simulink model "BlockDiagram"  (R2021a)
settings: Solver=VariableStepAuto  StartTime=0.0  StopTime=10.0  RelTol=1e-3
values from neighbouring files (symbols this model uses):
  a = 0    [gainMaxDef.m]    (also in plot2.m = 2; simulink_test.m = 5)
  alpha = 1.195    [gainMaxDef.m]    (also in plot2.m = 1.9; simulink_test.m = 1.192)
  betac = 2    [plot2.m]    (also in simulink_test.m = 10)
  delay = 0.5    [plot2.m]    (also in simulink_test.m = 0.015)
  delay_a = 0.150    (= 0.15)    [plot2.m]    (also in simulink_test.m = 0.01)
  gnet = 40    [plot2.m]    (also in simulink_test.m = gnetset(k))
  omega = omegalist(l)    [gainMaxDef.m]    (also in plot2.m = 300; simulink_test.m = 0.8)
  omegader = 80    [simulink_test.m]
libraries: cstblocks x12
settings Model: Creator=shiva  LastModifiedBy=shiva

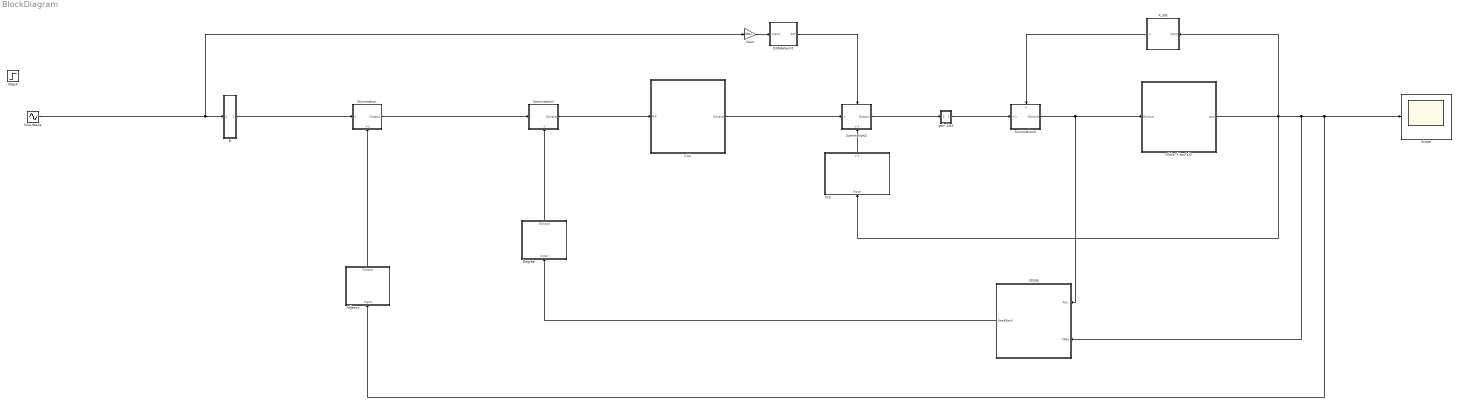
== system BlockDiagram ==
  Adjency : Subsystem
  B : Subsystem
  C(s) : Subsystem
  CDOB : Subsystem
  DSRdelayV2 : Subsystem
  Degree : Subsystem
  F(s) : Subsystem
  G(s)e^(-tau*s)2 : Subsystem
  Gain : Gain  Gain=betac
  Scope : Scope
  Sine Wave : Sin  SampleTime=0
  Step3 : Step  Time=0  SampleTime=0
  Summation : Subsystem
      settings: PortSchema="{\"entries\":[{\"content\":{\"sides\":[{\"content\":{\"connectorIds\":[\"In1\"]},\"type\":\"ConnectorPlacement.EquallySpacedRectSide\",\"uuid\":\"34a8278e-9c45-4ba9-8e7e-23ce47585cde\"},{\"content\":{\"connectorIds\":[\"Out1\"],\"side\":\"RIGHT\"},\"type\":\"ConnectorPlacement.EquallySpacedRectSide\",\"uuid\":\"649ea4d6-7388-43bb-a9cc-df912747b53e\"},{\"content\":{\"connectorIds\":[],\"side\":\"TOP\"},\"type\":\"ConnectorPlacement.EquallySpacedRectSide\",\"uuid\":\"5c1b8a35-4e2e-4e66-a4c8-170892603f16\"},{\"content\":{\"connectorIds\":[\"In2\"],\"side\":\"BOTTOM\"},\"type\":\"ConnectorPlacement.EquallySpacedRectSide\",\"uuid\":\"84c9cce4-2c6f-4c0c-8925-f02fa0e78f13\"}]},\"type\":\"ConnectorPlacement.EquallySpacedConnector\",\"uuid\":\"f49b62c2-1801-4f66-a651-2f339c5f1b03\"}],\"packageUris\":[\"http://schema.mathworks.com/mf0/Connector/R2020b\"],\"version\":\"1.0\"}"
  Summation1 : Subsystem
      settings: PortSchema="{\"entries\":[{\"content\":{\"sides\":[{\"content\":{\"connectorIds\":[\"In1\"]},\"type\":\"ConnectorPlacement.EquallySpacedRectSide\",\"uuid\":\"34a8278e-9c45-4ba9-8e7e-23ce47585cde\"},{\"content\":{\"connectorIds\":[\"Out1\"],\"side\":\"RIGHT\"},\"type\":\"ConnectorPlacement.EquallySpacedRectSide\",\"uuid\":\"649ea4d6-7388-43bb-a9cc-df912747b53e\"},{\"content\":{\"connectorIds\":[],\"side\":\"TOP\"},\"type\":\"ConnectorPlacement.EquallySpacedRectSide\",\"uuid\":\"5c1b8a35-4e2e-4e66-a4c8-170892603f16\"},{\"content\":{\"connectorIds\":[\"In2\"],\"side\":\"BOTTOM\"},\"type\":\"ConnectorPlacement.EquallySpacedRectSide\",\"uuid\":\"84c9cce4-2c6f-4c0c-8925-f02fa0e78f13\"}]},\"type\":\"ConnectorPlacement.EquallySpacedConnector\",\"uuid\":\"f49b62c2-1801-4f66-a651-2f339c5f1b03\"}],\"packageUris\":[\"http://schema.mathworks.com/mf0/Connector/R2020b\"],\"version\":\"1.0\"}"
  Summation2 : Subsystem
      settings: PortSchema="{\"entries\":[{\"content\":{\"sides\":[{\"content\":{\"connectorIds\":[\"In1\"]},\"type\":\"ConnectorPlacement.EquallySpacedRectSide\",\"uuid\":\"34a8278e-9c45-4ba9-8e7e-23ce47585cde\"},{\"content\":{\"connectorIds\":[\"Out1\"],\"side\":\"RIGHT\"},\"type\":\"ConnectorPlacement.EquallySpacedRectSide\",\"uuid\":\"649ea4d6-7388-43bb-a9cc-df912747b53e\"},{\"content\":{\"connectorIds\":[\"In2\"],\"side\":\"TOP\"},\"type\":\"ConnectorPlacement.EquallySpacedRectSide\",\"uuid\":\"5c1b8a35-4e2e-4e66-a4c8-170892603f16\"},{\"content\":{\"connectorIds\":[\"In3\"],\"side\":\"BOTTOM\"},\"type\":\"ConnectorPlacement.EquallySpacedRectSide\",\"uuid\":\"84c9cce4-2c6f-4c0c-8925-f02fa0e78f13\"}]},\"type\":\"ConnectorPlacement.EquallySpacedConnector\",\"uuid\":\"f49b62c2-1801-4f66-a651-2f339c5f1b03\"}],\"packageUris\":[\"http://schema.mathworks.com/mf0/Connector/R2020b\"],\"version\":\"1.0\"}"
  Summation3 : Subsystem
      settings: PortSchema="{\"entries\":[{\"content\":{\"sides\":[{\"content\":{\"connectorIds\":[\"In1\"]},\"type\":\"ConnectorPlacement.EquallySpacedRectSide\",\"uuid\":\"34a8278e-9c45-4ba9-8e7e-23ce47585cde\"},{\"content\":{\"connectorIds\":[\"Out1\"],\"side\":\"RIGHT\"},\"type\":\"ConnectorPlacement.EquallySpacedRectSide\",\"uuid\":\"649ea4d6-7388-43bb-a9cc-df912747b53e\"},{\"content\":{\"connectorIds\":[\"In2\"],\"side\":\"TOP\"},\"type\":\"ConnectorPlacement.EquallySpacedRectSide\",\"uuid\":\"5c1b8a35-4e2e-4e66-a4c8-170892603f16\"},{\"content\":{\"connectorIds\":[],\"side\":\"BOTTOM\"},\"type\":\"ConnectorPlacement.EquallySpacedRectSide\",\"uuid\":\"84c9cce4-2c6f-4c0c-8925-f02fa0e78f13\"}]},\"type\":\"ConnectorPlacement.EquallySpacedConnector\",\"uuid\":\"f49b62c2-1801-4f66-a651-2f339c5f1b03\"}],\"packageUris\":[\"http://schema.mathworks.com/mf0/Connector/R2020b\"],\"version\":\"1.0\"}"
  X_dot : Subsystem
  gain 1/a2 : Subsystem
  wires:
  Gain/1 -> DSRdelayV2/1(Input)
  Sine Wave/1 -> Gain/1, B/1(Input)
  G(s)e^(-tau*s)2/1(pos) -> F(s)/1(Input), CDOB/2(XRes), Adjency/1(Input), Scope/1, X_dot/1(Input)
  B/1(Output) -> Summation/1(+)
  gain 1/a2/1(u/a) -> Summation3/1(+1)
  X_dot/1(+) -> Summation3/2(+)
  Summation3/1(Output) -> CDOB/1(Acc.), G(s)e^(-tau*s)2/1(Output)
  Summation2/1(Output) -> gain 1/a2/1(u)
  F(s)/1(+1) -> Summation2/3(+1)
  DSRdelayV2/1(est) -> Summation2/2(-)
  C(s)/1(Output) -> Summation2/1(+)
  Summation1/1(Output) -> C(s)/1(R-F)
  Degree/1(Output) -> Summation1/2(+)
  Adjency/1(Output) -> Summation/2(+1)
  Summation/1(Output) -> Summation1/1(-)
  CDOB/1(FeedBack) -> Degree/1(Input)

== system BlockDiagram/Adjency ==
  Input : Inport
  Demux : Demux  Outputs=6
  Mux : Mux  Inputs=6
  Sum : Sum  Inputs=|++
  Sum1 : Sum  Inputs=|++
  Sum2 : Sum  Inputs=++++
  Terminator : Terminator
  Zero : Constant  Value=0  OutDataTypeStr=Inherit: Inherit via back propagation
  Output : Outport
  wires:
  Demux/2 -> Sum2/1, Mux/4, Sum1/2
  Demux/4 -> Sum2/3
  Demux/1 -> Sum1/1, Sum/1
  Sum1/1 -> Mux/3
  Zero/1 -> Mux/1
  Demux/6 -> Terminator/1
  Sum2/1 -> Mux/6
  Sum/1 -> Mux/2
  Demux/5 -> Sum2/4
  Demux/3 -> Sum/2, Mux/5, Sum2/2
  Input/1 -> Demux/1
  Mux/1 -> Output/1

== system BlockDiagram/B ==
  Input : Inport
  Mux : Mux  Inputs=6
  Zero : Constant  Value=0  OutDataTypeStr=Inherit: Inherit via back propagation
  Output : Outport
  wires:
  Input/1 -> Mux/1
  Zero/1 -> Mux/6, Mux/5, Mux/3, Mux/2, Mux/4
  Mux/1 -> Output/1

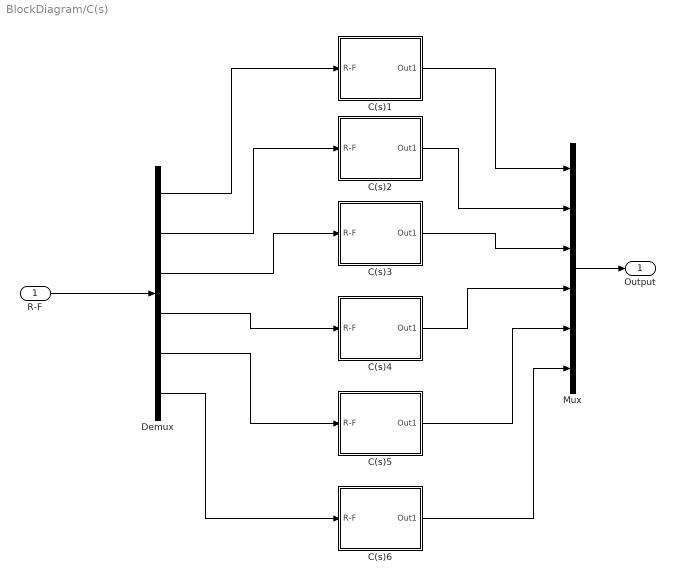
== system BlockDiagram/C(s) ==
  R-F : Inport
  C(s)1 : Subsystem
  C(s)2 : Subsystem
  C(s)3 : Subsystem
  C(s)4 : Subsystem
  C(s)5 : Subsystem
  C(s)6 : Subsystem
  Demux : Demux  Outputs=6
  Mux : Mux  Inputs=6
  Output : Outport
  wires:
  Demux/1 -> C(s)1/1(R-F)
  Demux/2 -> C(s)2/1(R-F)
  Demux/3 -> C(s)3/1(R-F)
  Demux/4 -> C(s)4/1(R-F)
  Demux/5 -> C(s)5/1(R-F)
  Demux/6 -> C(s)6/1(R-F)
  Mux/1 -> Output/1
  R-F/1 -> Demux/1
  C(s)1/1(Out1) -> Mux/1
  C(s)2/1(Out1) -> Mux/2
  C(s)3/1(Out1) -> Mux/3
  C(s)4/1(Out1) -> Mux/4
  C(s)5/1(Out1) -> Mux/5
  C(s)6/1(Out1) -> Mux/6

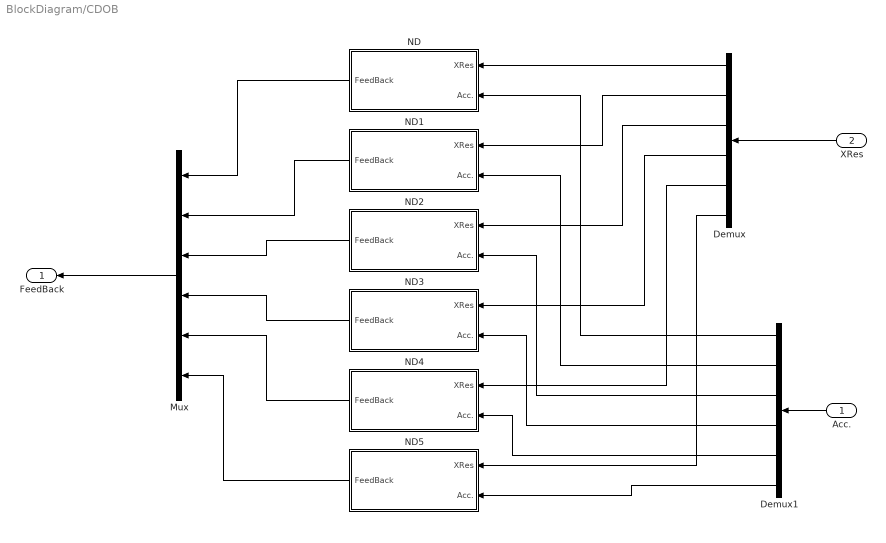
== system BlockDiagram/CDOB ==
  Acc. : Inport
  XRes : Inport  Port=2
  Demux : Demux  Outputs=6
  Demux1 : Demux  Outputs=6
  Mux : Mux  Inputs=6
  ND : Subsystem
  ND1 : Subsystem
  ND2 : Subsystem
  ND3 : Subsystem
  ND4 : Subsystem
  ND5 : Subsystem
  FeedBack : Outport
  wires:
  ND5/1(FeedBack) -> Mux/6
  ND1/1(FeedBack) -> Mux/2
  ND2/1(FeedBack) -> Mux/3
  ND4/1(FeedBack) -> Mux/5
  ND3/1(FeedBack) -> Mux/4
  ND/1(FeedBack) -> Mux/1
  Mux/1 -> FeedBack/1
  Demux/1 -> ND/1(XRes)
  Demux/2 -> ND1/1(XRes)
  Demux/3 -> ND2/1(XRes)
  Demux/4 -> ND3/1(XRes)
  Demux/5 -> ND4/1(XRes)
  Demux1/1 -> ND/2(Acc.)
  Demux1/2 -> ND1/2(Acc.)
  Demux1/3 -> ND2/2(Acc.)
  Demux1/4 -> ND3/2(Acc.)
  Demux1/5 -> ND4/2(Acc.)
  Acc./1 -> Demux1/1
  XRes/1 -> Demux/1
  Demux1/6 -> ND5/2(Acc.)
  Demux/6 -> ND5/1(XRes)

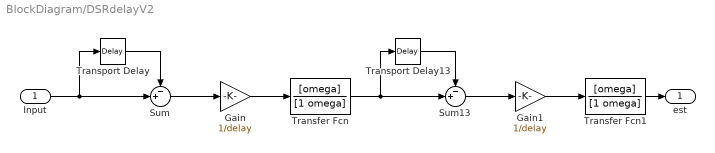
== system BlockDiagram/DSRdelayV2 ==
  Input : Inport
  Gain : Gain  Gain=1/delay
  Gain1 : Gain  Gain=1/delay
  Sum : Sum  Inputs=-+|
  Sum13 : Sum  Inputs=-+|
  Transfer Fcn : TransferFcn  Numerator=[omega]  Denominator=[1 omega]
  Transfer Fcn1 : TransferFcn  Numerator=[omega]  Denominator=[1 omega]
  Transport Delay : TransportDelay  DelayTime=delay
  Transport Delay13 : TransportDelay  DelayTime=delay
  est : Outport
  wires:
  Sum/1 -> Gain/1
  Gain/1 -> Transfer Fcn/1
  Transfer Fcn/1 -> Transport Delay13/1, Sum13/2
  Input/1 -> Transport Delay/1, Sum/2
  Transport Delay/1 -> Sum/1
  Transfer Fcn1/1 -> est/1
  Transport Delay13/1 -> Sum13/1
  Gain1/1 -> Transfer Fcn1/1
  Sum13/1 -> Gain1/1

== system BlockDiagram/Degree ==
  Input : Inport
  Demux : Demux  Outputs=6
  Gain : Gain  Gain=2
  Gain1 : Gain  Gain=2
  Gain4 : Gain  Gain=4
  Mux : Mux  Inputs=6
  Output : Outport
  wires:
  Gain1/1 -> Mux/3
  Demux/6 -> Gain4/1
  Gain4/1 -> Mux/6
  Gain/1 -> Mux/2
  Mux/1 -> Output/1
  Demux/1 -> Mux/1
  Demux/2 -> Gain/1
  Demux/3 -> Gain1/1
  Demux/4 -> Mux/4
  Demux/5 -> Mux/5
  Input/1 -> Demux/1

== system BlockDiagram/F(s) ==
  Input : Inport
  DSRdelayV1 : Subsystem
  DSRdelayV2 : Subsystem
  DSRdelayV3 : Subsystem
  DSRdelayV4 : Subsystem
  DSRdelayV5 : Subsystem
  DSRdelayV6 : Subsystem
  Demux : Demux  Outputs=6
  Mux : Mux  Inputs=6
  +1 : Outport
  wires:
  Input/1 -> Demux/1
  Mux/1 -> +1/1
  Demux/1 -> DSRdelayV2/1(Input)
  Demux/2 -> DSRdelayV1/1(Input)
  Demux/3 -> DSRdelayV3/1(Input)
  Demux/4 -> DSRdelayV4/1(Input)
  Demux/5 -> DSRdelayV5/1(Input)
  Demux/6 -> DSRdelayV6/1(Input)
  DSRdelayV2/1(est) -> Mux/1
  DSRdelayV1/1(est) -> Mux/2
  DSRdelayV3/1(est) -> Mux/3
  DSRdelayV4/1(est) -> Mux/4
  DSRdelayV5/1(est) -> Mux/5
  DSRdelayV6/1(est) -> Mux/6

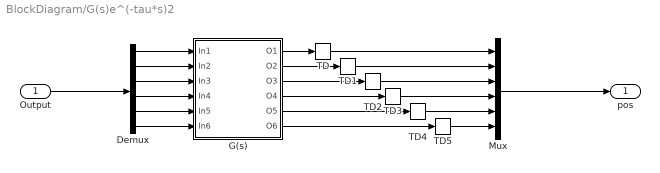
== system BlockDiagram/G(s)e^(-tau*s)2 ==
  Output : Inport
  Demux : Demux  Outputs=6
  G(s) : Subsystem
  Mux : Mux  Inputs=6
  TD{,1..5} (6 alike) : TransportDelay  DelayTime=delay_a
  pos : Outport
  wires:
  G(s)/3(O3) -> TD2/1
  G(s)/1(O1) -> TD/1
  G(s)/4(O4) -> TD3/1
  G(s)/5(O5) -> TD4/1
  G(s)/6(O6) -> TD5/1
  G(s)/2(O2) -> TD1/1
  Demux/1 -> G(s)/1(In1)
  Demux/2 -> G(s)/2(In2)
  Demux/3 -> G(s)/3(In3)
  Demux/4 -> G(s)/4(In4)
  Demux/5 -> G(s)/5(In5)
  Demux/6 -> G(s)/6(In6)
  Output/1 -> Demux/1
  TD/1 -> Mux/1
  Mux/1 -> pos/1
  TD1/1 -> Mux/2
  TD2/1 -> Mux/3
  TD3/1 -> Mux/4
  TD4/1 -> Mux/5
  TD5/1 -> Mux/6

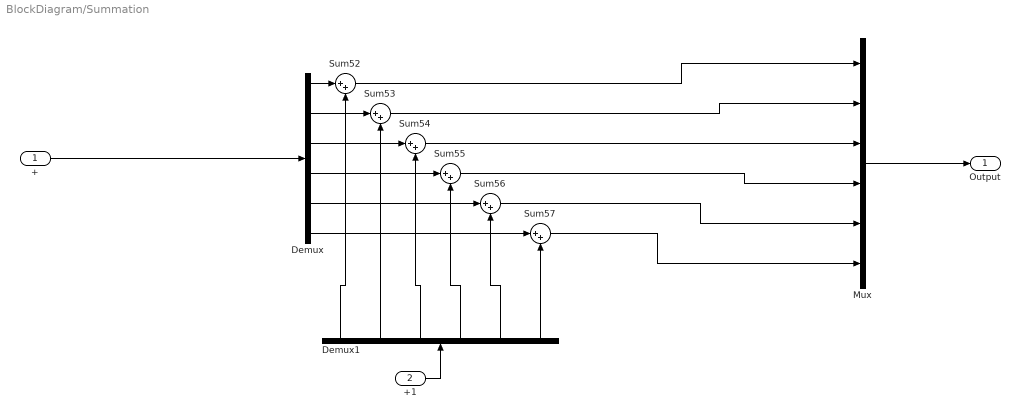
== system BlockDiagram/Summation ==
  + : Inport
  +1 : Inport  Port=2
  Demux : Demux  Outputs=6
  Demux1 : Demux  Outputs=6
  Mux : Mux  Inputs=6
  Sum{52..57} (6 alike) : Sum  Inputs=|++
  Output : Outport
  wires:
  Demux/3 -> Sum54/1
  Sum57/1 -> Mux/6
  Demux1/4 -> Sum55/2
  Demux/4 -> Sum55/1
  Sum56/1 -> Mux/5
  Demux/2 -> Sum53/1
  Demux1/1 -> Sum52/2
  Demux1/5 -> Sum56/2
  Demux1/6 -> Sum57/2
  Demux/6 -> Sum57/1
  Sum54/1 -> Mux/3
  Demux/5 -> Sum56/1
  Demux1/3 -> Sum54/2
  Demux/1 -> Sum52/1
  Demux1/2 -> Sum53/2
  +/1 -> Demux/1
  +1/1 -> Demux1/1
  Sum52/1 -> Mux/1
  Sum53/1 -> Mux/2
  Sum55/1 -> Mux/4
  Mux/1 -> Output/1

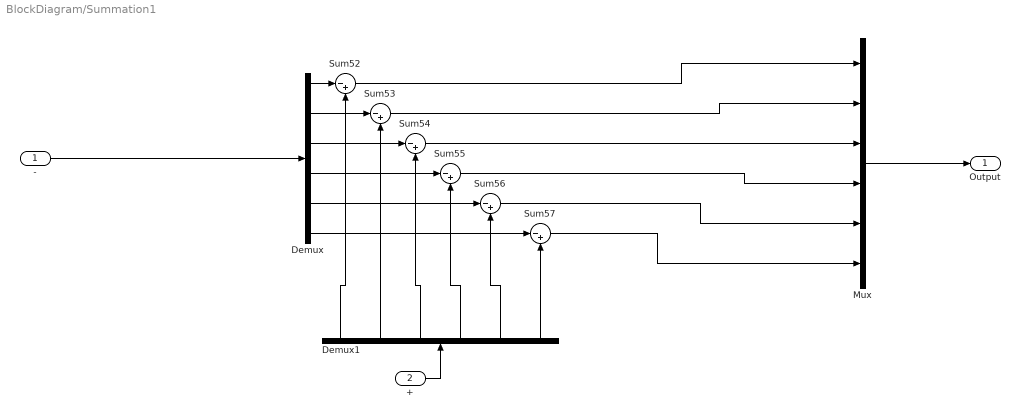
== system BlockDiagram/Summation1 ==
  - : Inport
  + : Inport  Port=2
  Demux : Demux  Outputs=6
  Demux1 : Demux  Outputs=6
  Mux : Mux  Inputs=6
  Sum{52..57} (6 alike) : Sum  Inputs=|-+
  Output : Outport
  wires:
  Demux/3 -> Sum54/1
  Sum57/1 -> Mux/6
  Demux1/4 -> Sum55/2
  Demux/4 -> Sum55/1
  Sum56/1 -> Mux/5
  Demux/2 -> Sum53/1
  Demux1/1 -> Sum52/2
  Demux1/5 -> Sum56/2
  Demux1/6 -> Sum57/2
  Demux/6 -> Sum57/1
  Sum54/1 -> Mux/3
  Demux/5 -> Sum56/1
  Demux1/3 -> Sum54/2
  Demux/1 -> Sum52/1
  Demux1/2 -> Sum53/2
  -/1 -> Demux/1
  +/1 -> Demux1/1
  Sum52/1 -> Mux/1
  Sum53/1 -> Mux/2
  Sum55/1 -> Mux/4
  Mux/1 -> Output/1

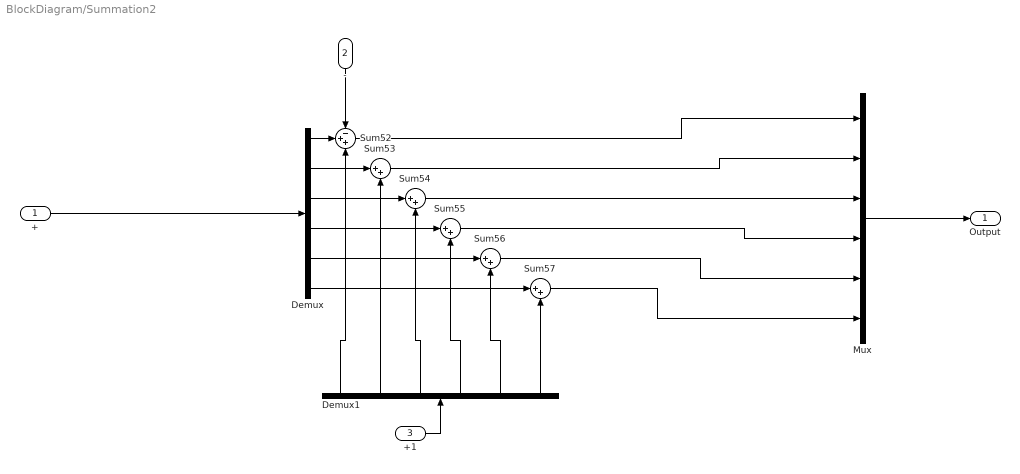
== system BlockDiagram/Summation2 ==
  + : Inport
  - : Inport  Port=2
  +1 : Inport  Port=3
  Demux : Demux  Outputs=6
  Demux1 : Demux  Outputs=6
  Mux : Mux  Inputs=6
  Sum52 : Sum  Inputs=-++
  Sum{53..57} (5 alike) : Sum  Inputs=|++
  Output : Outport
  wires:
  Demux/3 -> Sum54/1
  Sum57/1 -> Mux/6
  Demux1/4 -> Sum55/2
  Demux/4 -> Sum55/1
  Sum56/1 -> Mux/5
  Demux/2 -> Sum53/1
  Demux1/5 -> Sum56/2
  Demux1/6 -> Sum57/2
  Demux/6 -> Sum57/1
  Sum54/1 -> Mux/3
  Demux/5 -> Sum56/1
  Demux1/3 -> Sum54/2
  Demux1/2 -> Sum53/2
  +/1 -> Demux/1
  +1/1 -> Demux1/1
  Sum52/1 -> Mux/1
  Sum53/1 -> Mux/2
  Sum55/1 -> Mux/4
  Mux/1 -> Output/1
  Demux/1 -> Sum52/2
  -/1 -> Sum52/1
  Demux1/1 -> Sum52/3

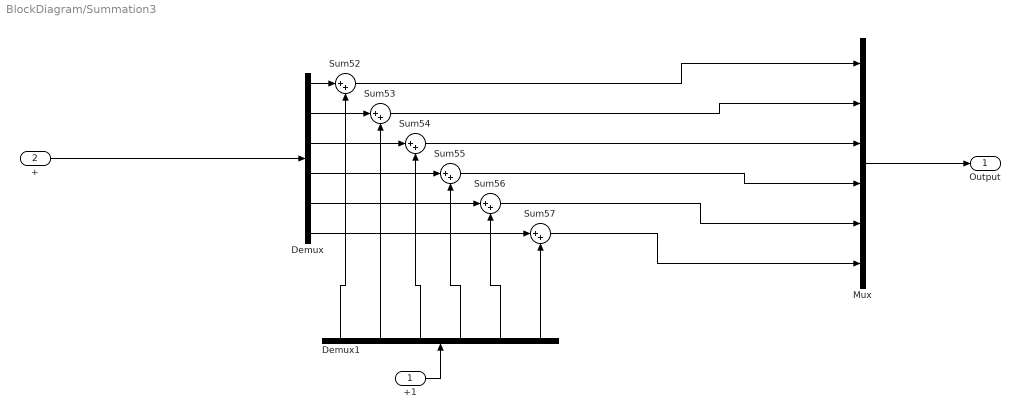
== system BlockDiagram/Summation3 ==
  +1 : Inport
  + : Inport  Port=2
  Demux : Demux  Outputs=6
  Demux1 : Demux  Outputs=6
  Mux : Mux  Inputs=6
  Sum{52..57} (6 alike) : Sum  Inputs=|++
  Output : Outport
  wires:
  Demux/3 -> Sum54/1
  Sum57/1 -> Mux/6
  Demux1/4 -> Sum55/2
  Demux/4 -> Sum55/1
  Sum56/1 -> Mux/5
  Demux/2 -> Sum53/1
  Demux1/1 -> Sum52/2
  Demux1/5 -> Sum56/2
  Demux1/6 -> Sum57/2
  Demux/6 -> Sum57/1
  Sum54/1 -> Mux/3
  Demux/5 -> Sum56/1
  Demux1/3 -> Sum54/2
  Demux/1 -> Sum52/1
  Demux1/2 -> Sum53/2
  +/1 -> Demux/1
  +1/1 -> Demux1/1
  Sum52/1 -> Mux/1
  Sum53/1 -> Mux/2
  Sum55/1 -> Mux/4
  Mux/1 -> Output/1

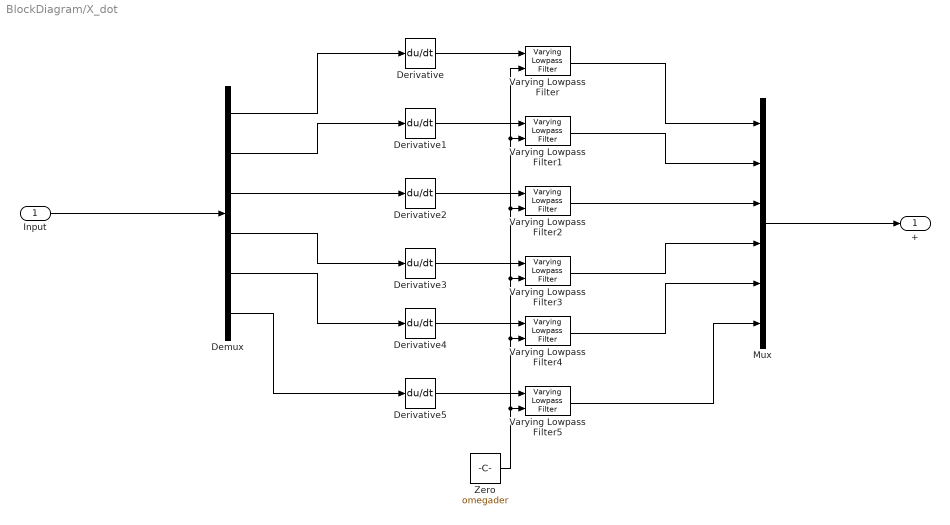
== system BlockDiagram/X_dot ==
  Input : Inport
  Demux : Demux  Outputs=6
  Derivative{,1..5} (6 alike) : Derivative
  Mux : Mux  Inputs=6
  Varying Lowpass Filter{,1..5} (6 alike) : cstblocks/Linear Parameter Varying/Varying Lowpass Filter  N=1
  Zero : Constant  Value=omegader  OutDataTypeStr=Inherit: Inherit via back propagation
  + : Outport
  wires:
  Derivative/1 -> Varying Lowpass Filter/1
  Derivative1/1 -> Varying Lowpass Filter1/1
  Derivative2/1 -> Varying Lowpass Filter2/1
  Derivative3/1 -> Varying Lowpass Filter3/1
  Derivative4/1 -> Varying Lowpass Filter4/1
  Derivative5/1 -> Varying Lowpass Filter5/1
  Zero/1 -> Varying Lowpass Filter3/2, Varying Lowpass Filter/2, Varying Lowpass Filter1/2, Varying Lowpass Filter2/2, Varying Lowpass Filter4/2, Varying Lowpass Filter5/2
  Input/1 -> Demux/1
  Demux/1 -> Derivative/1
  Demux/2 -> Derivative1/1
  Demux/3 -> Derivative2/1
  Demux/4 -> Derivative3/1
  Demux/5 -> Derivative4/1
  Demux/6 -> Derivative5/1
  Varying Lowpass Filter2/1 -> Mux/3
  Varying Lowpass Filter1/1 -> Mux/2
  Varying Lowpass Filter/1 -> Mux/1
  Varying Lowpass Filter3/1 -> Mux/4
  Varying Lowpass Filter4/1 -> Mux/5
  Varying Lowpass Filter5/1 -> Mux/6
  Mux/1 -> +/1

== system BlockDiagram/gain 1//a2 ==
  u : Inport
  1/a{,1..5} (6 alike) : Gain  Gain=1/a
  Demux : Demux  Outputs=6
  Mux : Mux  Inputs=6
  u/a : Outport
  wires:
  Mux/1 -> u/a/1
  u/1 -> Demux/1
  Demux/1 -> 1/a/1
  Demux/2 -> 1/a1/1
  Demux/3 -> 1/a2/1
  Demux/4 -> 1/a3/1
  Demux/5 -> 1/a4/1
  Demux/6 -> 1/a5/1
  1/a/1 -> Mux/1
  1/a1/1 -> Mux/2
  1/a2/1 -> Mux/3
  1/a3/1 -> Mux/4
  1/a4/1 -> Mux/5
  1/a5/1 -> Mux/6

== system BlockDiagram/C(s)/C(s)1 ==
  R-F : Inport
  DSRdelayV1 : Subsystem
  Derivative : Derivative
  Gain : Gain  Gain=betac
  Gain1 : Gain  Gain=betac*alpha^2
  Gain3 : Gain  Gain=2*alpha*betac
  Sum : Sum  Inputs=---
  Varying Lowpass Filter : cstblocks/Linear Parameter Varying/Varying Lowpass Filter  N=1
  Zero : Constant  Value=omegader  OutDataTypeStr=Inherit: Inherit via back propagation
  Out1 : Outport
  wires:
  Gain/1 -> DSRdelayV1/1(Input)
  Gain1/1 -> Sum/2
  Sum/1 -> Out1/1
  R-F/1 -> Gain3/1, Gain1/1, Gain/1
  DSRdelayV1/1(est) -> Sum/1
  Zero/1 -> Varying Lowpass Filter/2
  Varying Lowpass Filter/1 -> Sum/3
  Gain3/1 -> Derivative/1
  Derivative/1 -> Varying Lowpass Filter/1

== system BlockDiagram/C(s)/C(s)2 ==
  R-F : Inport
  DSRdelayV1 : Subsystem
  Derivative : Derivative
  Gain : Gain  Gain=betac
  Gain1 : Gain  Gain=betac*alpha^2
  Gain3 : Gain  Gain=2*alpha*betac
  Sum : Sum  Inputs=---
  Varying Lowpass Filter : cstblocks/Linear Parameter Varying/Varying Lowpass Filter  N=1
  Zero : Constant  Value=omegader  OutDataTypeStr=Inherit: Inherit via back propagation
  Out1 : Outport
  wires:
  Gain/1 -> DSRdelayV1/1(Input)
  Gain1/1 -> Sum/2
  Sum/1 -> Out1/1
  R-F/1 -> Gain3/1, Gain1/1, Gain/1
  DSRdelayV1/1(est) -> Sum/1
  Zero/1 -> Varying Lowpass Filter/2
  Varying Lowpass Filter/1 -> Sum/3
  Gain3/1 -> Derivative/1
  Derivative/1 -> Varying Lowpass Filter/1

== system BlockDiagram/C(s)/C(s)3 ==
  R-F : Inport
  DSRdelayV1 : Subsystem
  Derivative : Derivative
  Gain : Gain  Gain=betac
  Gain1 : Gain  Gain=betac*alpha^2
  Gain3 : Gain  Gain=2*alpha*betac
  Sum : Sum  Inputs=---
  Varying Lowpass Filter : cstblocks/Linear Parameter Varying/Varying Lowpass Filter  N=1
  Zero : Constant  Value=omegader  OutDataTypeStr=Inherit: Inherit via back propagation
  Out1 : Outport
  wires:
  Gain/1 -> DSRdelayV1/1(Input)
  Gain1/1 -> Sum/2
  Sum/1 -> Out1/1
  R-F/1 -> Gain3/1, Gain1/1, Gain/1
  DSRdelayV1/1(est) -> Sum/1
  Zero/1 -> Varying Lowpass Filter/2
  Varying Lowpass Filter/1 -> Sum/3
  Gain3/1 -> Derivative/1
  Derivative/1 -> Varying Lowpass Filter/1

== system BlockDiagram/C(s)/C(s)4 ==
  R-F : Inport
  DSRdelayV1 : Subsystem
  Derivative : Derivative
  Gain : Gain  Gain=betac
  Gain1 : Gain  Gain=betac*alpha^2
  Gain3 : Gain  Gain=2*alpha*betac
  Sum : Sum  Inputs=---
  Varying Lowpass Filter : cstblocks/Linear Parameter Varying/Varying Lowpass Filter  N=1
  Zero : Constant  Value=omegader  OutDataTypeStr=Inherit: Inherit via back propagation
  Out1 : Outport
  wires:
  Gain/1 -> DSRdelayV1/1(Input)
  Gain1/1 -> Sum/2
  Sum/1 -> Out1/1
  R-F/1 -> Gain3/1, Gain1/1, Gain/1
  DSRdelayV1/1(est) -> Sum/1
  Zero/1 -> Varying Lowpass Filter/2
  Varying Lowpass Filter/1 -> Sum/3
  Gain3/1 -> Derivative/1
  Derivative/1 -> Varying Lowpass Filter/1

== system BlockDiagram/C(s)/C(s)5 ==
  R-F : Inport
  DSRdelayV1 : Subsystem
  Derivative : Derivative
  Gain : Gain  Gain=betac
  Gain1 : Gain  Gain=betac*alpha^2
  Gain3 : Gain  Gain=2*alpha*betac
  Sum : Sum  Inputs=---
  Varying Lowpass Filter : cstblocks/Linear Parameter Varying/Varying Lowpass Filter  N=1
  Zero : Constant  Value=omegader  OutDataTypeStr=Inherit: Inherit via back propagation
  Out1 : Outport
  wires:
  Gain/1 -> DSRdelayV1/1(Input)
  Gain1/1 -> Sum/2
  Sum/1 -> Out1/1
  R-F/1 -> Gain3/1, Gain1/1, Gain/1
  DSRdelayV1/1(est) -> Sum/1
  Zero/1 -> Varying Lowpass Filter/2
  Varying Lowpass Filter/1 -> Sum/3
  Gain3/1 -> Derivative/1
  Derivative/1 -> Varying Lowpass Filter/1

== system BlockDiagram/C(s)/C(s)6 ==
  R-F : Inport
  DSRdelayV1 : Subsystem
  Derivative : Derivative
  Gain : Gain  Gain=betac
  Gain1 : Gain  Gain=betac*alpha^2
  Gain3 : Gain  Gain=2*alpha*betac
  Sum : Sum  Inputs=---
  Varying Lowpass Filter : cstblocks/Linear Parameter Varying/Varying Lowpass Filter  N=1
  Zero : Constant  Value=omegader  OutDataTypeStr=Inherit: Inherit via back propagation
  Out1 : Outport
  wires:
  Gain/1 -> DSRdelayV1/1(Input)
  Gain1/1 -> Sum/2
  Sum/1 -> Out1/1
  R-F/1 -> Gain3/1, Gain1/1, Gain/1
  DSRdelayV1/1(est) -> Sum/1
  Zero/1 -> Varying Lowpass Filter/2
  Varying Lowpass Filter/1 -> Sum/3
  Gain3/1 -> Derivative/1
  Derivative/1 -> Varying Lowpass Filter/1

== system BlockDiagram/CDOB/ND ==
  XRes : Inport
  Acc. : Inport  Port=2
  CDOB1 : Subsystem
  TimeDelayComp : Subsystem
  FeedBack : Outport
  wires:
  CDOB1/1(Dobsv) -> TimeDelayComp/2(Dobsv)
  Acc./1 -> CDOB1/2(Acc.)
  TimeDelayComp/1(FeedBack) -> FeedBack/1
  XRes/1 -> TimeDelayComp/1(SysOut), CDOB1/1(XRes)

== system BlockDiagram/CDOB/ND1 ==
  XRes : Inport
  Acc. : Inport  Port=2
  CDOB1 : Subsystem
  TimeDelayComp : Subsystem
  FeedBack : Outport
  wires:
  CDOB1/1(Dobsv) -> TimeDelayComp/2(Dobsv)
  Acc./1 -> CDOB1/2(Acc.)
  TimeDelayComp/1(FeedBack) -> FeedBack/1
  XRes/1 -> TimeDelayComp/1(SysOut), CDOB1/1(XRes)

== system BlockDiagram/CDOB/ND2 ==
  XRes : Inport
  Acc. : Inport  Port=2
  CDOB1 : Subsystem
  TimeDelayComp : Subsystem
  FeedBack : Outport
  wires:
  CDOB1/1(Dobsv) -> TimeDelayComp/2(Dobsv)
  Acc./1 -> CDOB1/2(Acc.)
  TimeDelayComp/1(FeedBack) -> FeedBack/1
  XRes/1 -> TimeDelayComp/1(SysOut), CDOB1/1(XRes)

== system BlockDiagram/CDOB/ND3 ==
  XRes : Inport
  Acc. : Inport  Port=2
  CDOB1 : Subsystem
  TimeDelayComp : Subsystem
  FeedBack : Outport
  wires:
  CDOB1/1(Dobsv) -> TimeDelayComp/2(Dobsv)
  Acc./1 -> CDOB1/2(Acc.)
  TimeDelayComp/1(FeedBack) -> FeedBack/1
  XRes/1 -> TimeDelayComp/1(SysOut), CDOB1/1(XRes)

== system BlockDiagram/CDOB/ND4 ==
  XRes : Inport
  Acc. : Inport  Port=2
  CDOB1 : Subsystem
  TimeDelayComp : Subsystem
  FeedBack : Outport
  wires:
  CDOB1/1(Dobsv) -> TimeDelayComp/2(Dobsv)
  Acc./1 -> CDOB1/2(Acc.)
  TimeDelayComp/1(FeedBack) -> FeedBack/1
  XRes/1 -> TimeDelayComp/1(SysOut), CDOB1/1(XRes)

== system BlockDiagram/CDOB/ND5 ==
  XRes : Inport
  Acc. : Inport  Port=2
  CDOB1 : Subsystem
  TimeDelayComp : Subsystem
  FeedBack : Outport
  wires:
  CDOB1/1(Dobsv) -> TimeDelayComp/2(Dobsv)
  Acc./1 -> CDOB1/2(Acc.)
  TimeDelayComp/1(FeedBack) -> FeedBack/1
  XRes/1 -> TimeDelayComp/1(SysOut), CDOB1/1(XRes)

== system BlockDiagram/F(s)/DSRdelayV1 ==
  Input : Inport
  Gain : Gain  Gain=1/delay
  Gain1 : Gain  Gain=1/delay
  Sum : Sum  Inputs=-+|
  Sum13 : Sum  Inputs=-+|
  Transfer Fcn : TransferFcn  Numerator=[omega]  Denominator=[1 omega]
  Transfer Fcn1 : TransferFcn  Numerator=[omega]  Denominator=[1 omega]
  Transport Delay : TransportDelay  DelayTime=delay
  Transport Delay13 : TransportDelay  DelayTime=delay
  est : Outport
  wires:
  Sum/1 -> Gain/1
  Gain/1 -> Transfer Fcn/1
  Transfer Fcn/1 -> Transport Delay13/1, Sum13/2
  Input/1 -> Transport Delay/1, Sum/2
  Transport Delay/1 -> Sum/1
  Transfer Fcn1/1 -> est/1
  Transport Delay13/1 -> Sum13/1
  Gain1/1 -> Transfer Fcn1/1
  Sum13/1 -> Gain1/1

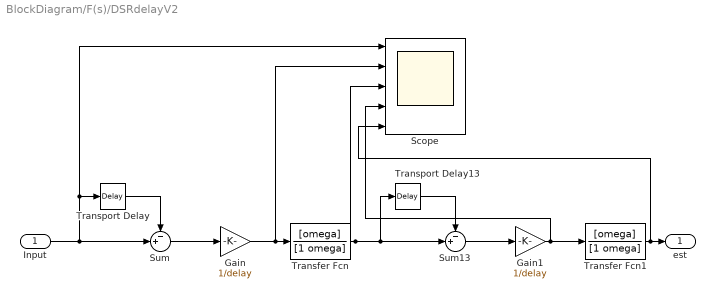
== system BlockDiagram/F(s)/DSRdelayV2 ==
  Input : Inport
  Gain : Gain  Gain=1/delay
  Gain1 : Gain  Gain=1/delay
  Scope : Scope  NumInputPorts=5
  Sum : Sum  Inputs=-+|
  Sum13 : Sum  Inputs=-+|
  Transfer Fcn : TransferFcn  Numerator=[omega]  Denominator=[1 omega]
  Transfer Fcn1 : TransferFcn  Numerator=[omega]  Denominator=[1 omega]
  Transport Delay : TransportDelay  DelayTime=delay
  Transport Delay13 : TransportDelay  DelayTime=delay
  est : Outport
  wires:
  Sum/1 -> Gain/1
  Gain/1 -> Scope/2, Transfer Fcn/1
  Transfer Fcn/1 -> Transport Delay13/1, Sum13/2, Scope/3
  Input/1 -> Transport Delay/1, Scope/1, Sum/2
  Transport Delay/1 -> Sum/1
  Transfer Fcn1/1 -> Scope/5, est/1
  Transport Delay13/1 -> Sum13/1
  Gain1/1 -> Scope/4, Transfer Fcn1/1
  Sum13/1 -> Gain1/1

== system BlockDiagram/F(s)/DSRdelayV3 ==
  Input : Inport
  Gain : Gain  Gain=1/delay
  Gain1 : Gain  Gain=1/delay
  Sum : Sum  Inputs=-+|
  Sum13 : Sum  Inputs=-+|
  Transfer Fcn : TransferFcn  Numerator=[omega]  Denominator=[1 omega]
  Transfer Fcn1 : TransferFcn  Numerator=[omega]  Denominator=[1 omega]
  Transport Delay : TransportDelay  DelayTime=delay
  Transport Delay13 : TransportDelay  DelayTime=delay
  est : Outport
  wires:
  Sum/1 -> Gain/1
  Gain/1 -> Transfer Fcn/1
  Transfer Fcn/1 -> Transport Delay13/1, Sum13/2
  Input/1 -> Transport Delay/1, Sum/2
  Transport Delay/1 -> Sum/1
  Transfer Fcn1/1 -> est/1
  Transport Delay13/1 -> Sum13/1
  Gain1/1 -> Transfer Fcn1/1
  Sum13/1 -> Gain1/1

== system BlockDiagram/F(s)/DSRdelayV4 ==
  Input : Inport
  Gain : Gain  Gain=1/delay
  Gain1 : Gain  Gain=1/delay
  Sum : Sum  Inputs=-+|
  Sum13 : Sum  Inputs=-+|
  Transfer Fcn : TransferFcn  Numerator=[omega]  Denominator=[1 omega]
  Transfer Fcn1 : TransferFcn  Numerator=[omega]  Denominator=[1 omega]
  Transport Delay : TransportDelay  DelayTime=delay
  Transport Delay13 : TransportDelay  DelayTime=delay
  est : Outport
  wires:
  Sum/1 -> Gain/1
  Gain/1 -> Transfer Fcn/1
  Transfer Fcn/1 -> Transport Delay13/1, Sum13/2
  Input/1 -> Transport Delay/1, Sum/2
  Transport Delay/1 -> Sum/1
  Transfer Fcn1/1 -> est/1
  Transport Delay13/1 -> Sum13/1
  Gain1/1 -> Transfer Fcn1/1
  Sum13/1 -> Gain1/1

== system BlockDiagram/F(s)/DSRdelayV5 ==
  Input : Inport
  Gain : Gain  Gain=1/delay
  Gain1 : Gain  Gain=1/delay
  Sum : Sum  Inputs=-+|
  Sum13 : Sum  Inputs=-+|
  Transfer Fcn : TransferFcn  Numerator=[omega]  Denominator=[1 omega]
  Transfer Fcn1 : TransferFcn  Numerator=[omega]  Denominator=[1 omega]
  Transport Delay : TransportDelay  DelayTime=delay
  Transport Delay13 : TransportDelay  DelayTime=delay
  est : Outport
  wires:
  Sum/1 -> Gain/1
  Gain/1 -> Transfer Fcn/1
  Transfer Fcn/1 -> Transport Delay13/1, Sum13/2
  Input/1 -> Transport Delay/1, Sum/2
  Transport Delay/1 -> Sum/1
  Transfer Fcn1/1 -> est/1
  Transport Delay13/1 -> Sum13/1
  Gain1/1 -> Transfer Fcn1/1
  Sum13/1 -> Gain1/1

== system BlockDiagram/F(s)/DSRdelayV6 ==
  Input : Inport
  Gain : Gain  Gain=1/delay
  Gain1 : Gain  Gain=1/delay
  Sum : Sum  Inputs=-+|
  Sum13 : Sum  Inputs=-+|
  Transfer Fcn : TransferFcn  Numerator=[omega]  Denominator=[1 omega]
  Transfer Fcn1 : TransferFcn  Numerator=[omega]  Denominator=[1 omega]
  Transport Delay : TransportDelay  DelayTime=delay
  Transport Delay13 : TransportDelay  DelayTime=delay
  est : Outport
  wires:
  Sum/1 -> Gain/1
  Gain/1 -> Transfer Fcn/1
  Transfer Fcn/1 -> Transport Delay13/1, Sum13/2
  Input/1 -> Transport Delay/1, Sum/2
  Transport Delay/1 -> Sum/1
  Transfer Fcn1/1 -> est/1
  Transport Delay13/1 -> Sum13/1
  Gain1/1 -> Transfer Fcn1/1
  Sum13/1 -> Gain1/1

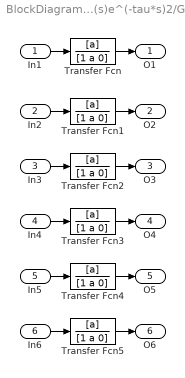
== system BlockDiagram/G(s)e^(-tau*s)2/G(s) ==
  In1 : Inport
  In2 : Inport  Port=2
  In3 : Inport  Port=3
  In4 : Inport  Port=4
  In5 : Inport  Port=5
  In6 : Inport  Port=6
  Transfer Fcn{,1..5} (6 alike) : TransferFcn  Numerator=[a]  Denominator=[1 a 0]
  O1 : Outport
  O2 : Outport  Port=2
  O3 : Outport  Port=3
  O4 : Outport  Port=4
  O5 : Outport  Port=5
  O6 : Outport  Port=6
  wires:
  Transfer Fcn1/1 -> O2/1
  In1/1 -> Transfer Fcn/1
  Transfer Fcn/1 -> O1/1
  In4/1 -> Transfer Fcn3/1
  Transfer Fcn3/1 -> O4/1
  In3/1 -> Transfer Fcn2/1
  In2/1 -> Transfer Fcn1/1
  Transfer Fcn2/1 -> O3/1
  Transfer Fcn5/1 -> O6/1
  In6/1 -> Transfer Fcn5/1
  In5/1 -> Transfer Fcn4/1
  Transfer Fcn4/1 -> O5/1

== system BlockDiagram/C(s)/C(s)1/DSRdelayV1 ==
  Input : Inport
  Gain : Gain  Gain=1/delay
  Gain1 : Gain  Gain=1/delay
  Sum : Sum  Inputs=-+|
  Sum13 : Sum  Inputs=-+|
  Transfer Fcn : TransferFcn  Numerator=[omega]  Denominator=[1 omega]
  Transfer Fcn1 : TransferFcn  Numerator=[omega]  Denominator=[1 omega]
  Transport Delay : TransportDelay  DelayTime=delay
  Transport Delay13 : TransportDelay  DelayTime=delay
  est : Outport
  wires:
  Sum/1 -> Gain/1
  Gain/1 -> Transfer Fcn/1
  Transfer Fcn/1 -> Transport Delay13/1, Sum13/2
  Input/1 -> Transport Delay/1, Sum/2
  Transport Delay/1 -> Sum/1
  Transfer Fcn1/1 -> est/1
  Transport Delay13/1 -> Sum13/1
  Gain1/1 -> Transfer Fcn1/1
  Sum13/1 -> Gain1/1

== system BlockDiagram/C(s)/C(s)2/DSRdelayV1 ==
  Input : Inport
  Gain : Gain  Gain=1/delay
  Gain1 : Gain  Gain=1/delay
  Sum : Sum  Inputs=-+|
  Sum13 : Sum  Inputs=-+|
  Transfer Fcn : TransferFcn  Numerator=[omega]  Denominator=[1 omega]
  Transfer Fcn1 : TransferFcn  Numerator=[omega]  Denominator=[1 omega]
  Transport Delay : TransportDelay  DelayTime=delay
  Transport Delay13 : TransportDelay  DelayTime=delay
  est : Outport
  wires:
  Sum/1 -> Gain/1
  Gain/1 -> Transfer Fcn/1
  Transfer Fcn/1 -> Transport Delay13/1, Sum13/2
  Input/1 -> Transport Delay/1, Sum/2
  Transport Delay/1 -> Sum/1
  Transfer Fcn1/1 -> est/1
  Transport Delay13/1 -> Sum13/1
  Gain1/1 -> Transfer Fcn1/1
  Sum13/1 -> Gain1/1

== system BlockDiagram/C(s)/C(s)3/DSRdelayV1 ==
  Input : Inport
  Gain : Gain  Gain=1/delay
  Gain1 : Gain  Gain=1/delay
  Sum : Sum  Inputs=-+|
  Sum13 : Sum  Inputs=-+|
  Transfer Fcn : TransferFcn  Numerator=[omega]  Denominator=[1 omega]
  Transfer Fcn1 : TransferFcn  Numerator=[omega]  Denominator=[1 omega]
  Transport Delay : TransportDelay  DelayTime=delay
  Transport Delay13 : TransportDelay  DelayTime=delay
  est : Outport
  wires:
  Sum/1 -> Gain/1
  Gain/1 -> Transfer Fcn/1
  Transfer Fcn/1 -> Transport Delay13/1, Sum13/2
  Input/1 -> Transport Delay/1, Sum/2
  Transport Delay/1 -> Sum/1
  Transfer Fcn1/1 -> est/1
  Transport Delay13/1 -> Sum13/1
  Gain1/1 -> Transfer Fcn1/1
  Sum13/1 -> Gain1/1

== system BlockDiagram/C(s)/C(s)4/DSRdelayV1 ==
  Input : Inport
  Gain : Gain  Gain=1/delay
  Gain1 : Gain  Gain=1/delay
  Sum : Sum  Inputs=-+|
  Sum13 : Sum  Inputs=-+|
  Transfer Fcn : TransferFcn  Numerator=[omega]  Denominator=[1 omega]
  Transfer Fcn1 : TransferFcn  Numerator=[omega]  Denominator=[1 omega]
  Transport Delay : TransportDelay  DelayTime=delay
  Transport Delay13 : TransportDelay  DelayTime=delay
  est : Outport
  wires:
  Sum/1 -> Gain/1
  Gain/1 -> Transfer Fcn/1
  Transfer Fcn/1 -> Transport Delay13/1, Sum13/2
  Input/1 -> Transport Delay/1, Sum/2
  Transport Delay/1 -> Sum/1
  Transfer Fcn1/1 -> est/1
  Transport Delay13/1 -> Sum13/1
  Gain1/1 -> Transfer Fcn1/1
  Sum13/1 -> Gain1/1

== system BlockDiagram/C(s)/C(s)5/DSRdelayV1 ==
  Input : Inport
  Gain : Gain  Gain=1/delay
  Gain1 : Gain  Gain=1/delay
  Sum : Sum  Inputs=-+|
  Sum13 : Sum  Inputs=-+|
  Transfer Fcn : TransferFcn  Numerator=[omega]  Denominator=[1 omega]
  Transfer Fcn1 : TransferFcn  Numerator=[omega]  Denominator=[1 omega]
  Transport Delay : TransportDelay  DelayTime=delay
  Transport Delay13 : TransportDelay  DelayTime=delay
  est : Outport
  wires:
  Sum/1 -> Gain/1
  Gain/1 -> Transfer Fcn/1
  Transfer Fcn/1 -> Transport Delay13/1, Sum13/2
  Input/1 -> Transport Delay/1, Sum/2
  Transport Delay/1 -> Sum/1
  Transfer Fcn1/1 -> est/1
  Transport Delay13/1 -> Sum13/1
  Gain1/1 -> Transfer Fcn1/1
  Sum13/1 -> Gain1/1

== system BlockDiagram/C(s)/C(s)6/DSRdelayV1 ==
  Input : Inport
  Gain : Gain  Gain=1/delay
  Gain1 : Gain  Gain=1/delay
  Sum : Sum  Inputs=-+|
  Sum13 : Sum  Inputs=-+|
  Transfer Fcn : TransferFcn  Numerator=[omega]  Denominator=[1 omega]
  Transfer Fcn1 : TransferFcn  Numerator=[omega]  Denominator=[1 omega]
  Transport Delay : TransportDelay  DelayTime=delay
  Transport Delay13 : TransportDelay  DelayTime=delay
  est : Outport
  wires:
  Sum/1 -> Gain/1
  Gain/1 -> Transfer Fcn/1
  Transfer Fcn/1 -> Transport Delay13/1, Sum13/2
  Input/1 -> Transport Delay/1, Sum/2
  Transport Delay/1 -> Sum/1
  Transfer Fcn1/1 -> est/1
  Transport Delay13/1 -> Sum13/1
  Gain1/1 -> Transfer Fcn1/1
  Sum13/1 -> Gain1/1

== system BlockDiagram/CDOB/ND/CDOB1 ==
  XRes : Inport
  Acc. : Inport  Port=2
  Derivative : Derivative  CoefficientInTFapproximation=0
  Gain : Gain  Gain=gnet/a
  Sum : Sum  Inputs=-+|
  Sum8 : Sum  Inputs=+-+
  Transfer Fcn2 : TransferFcn  Numerator=[gnet]  Denominator=[1 gnet]
  Dobsv : Outport
  wires:
  Transfer Fcn2/1 -> Sum/2
  Sum8/1 -> Transfer Fcn2/1
  Derivative/1 -> Sum8/2, Gain/1
  Gain/1 -> Sum8/1, Sum/1
  Sum/1 -> Dobsv/1
  XRes/1 -> Derivative/1
  Acc./1 -> Sum8/3

== system BlockDiagram/CDOB/ND/TimeDelayComp ==
  SysOut : Inport
  Dobsv : Inport  Port=2
  DelayCom : TransferFcn  Numerator=[a]  Denominator=[1 a 0]
  Sum8 : Sum  Inputs=|++
  FeedBack : Outport
  wires:
  DelayCom/1 -> Sum8/2
  SysOut/1 -> Sum8/1
  Sum8/1 -> FeedBack/1
  Dobsv/1 -> DelayCom/1

== system BlockDiagram/CDOB/ND1/CDOB1 ==
  XRes : Inport
  Acc. : Inport  Port=2
  Derivative : Derivative  CoefficientInTFapproximation=0
  Gain : Gain  Gain=gnet/a
  Sum : Sum  Inputs=-+|
  Sum8 : Sum  Inputs=+-+
  Transfer Fcn2 : TransferFcn  Numerator=[gnet]  Denominator=[1 gnet]
  Dobsv : Outport
  wires:
  Transfer Fcn2/1 -> Sum/2
  Sum8/1 -> Transfer Fcn2/1
  Derivative/1 -> Sum8/2, Gain/1
  Gain/1 -> Sum8/1, Sum/1
  Sum/1 -> Dobsv/1
  XRes/1 -> Derivative/1
  Acc./1 -> Sum8/3

== system BlockDiagram/CDOB/ND1/TimeDelayComp ==
  SysOut : Inport
  Dobsv : Inport  Port=2
  DelayCom : TransferFcn  Numerator=[a]  Denominator=[1 a 0]
  Sum8 : Sum  Inputs=|++
  FeedBack : Outport
  wires:
  DelayCom/1 -> Sum8/2
  SysOut/1 -> Sum8/1
  Sum8/1 -> FeedBack/1
  Dobsv/1 -> DelayCom/1

== system BlockDiagram/CDOB/ND2/CDOB1 ==
  XRes : Inport
  Acc. : Inport  Port=2
  Derivative : Derivative  CoefficientInTFapproximation=0
  Gain : Gain  Gain=gnet/a
  Sum : Sum  Inputs=-+|
  Sum8 : Sum  Inputs=+-+
  Transfer Fcn2 : TransferFcn  Numerator=[gnet]  Denominator=[1 gnet]
  Dobsv : Outport
  wires:
  Transfer Fcn2/1 -> Sum/2
  Sum8/1 -> Transfer Fcn2/1
  Derivative/1 -> Sum8/2, Gain/1
  Gain/1 -> Sum8/1, Sum/1
  Sum/1 -> Dobsv/1
  XRes/1 -> Derivative/1
  Acc./1 -> Sum8/3

== system BlockDiagram/CDOB/ND2/TimeDelayComp ==
  SysOut : Inport
  Dobsv : Inport  Port=2
  DelayCom : TransferFcn  Numerator=[a]  Denominator=[1 a 0]
  Sum8 : Sum  Inputs=|++
  FeedBack : Outport
  wires:
  DelayCom/1 -> Sum8/2
  SysOut/1 -> Sum8/1
  Sum8/1 -> FeedBack/1
  Dobsv/1 -> DelayCom/1

== system BlockDiagram/CDOB/ND3/CDOB1 ==
  XRes : Inport
  Acc. : Inport  Port=2
  Derivative : Derivative  CoefficientInTFapproximation=0
  Gain : Gain  Gain=gnet/a
  Sum : Sum  Inputs=-+|
  Sum8 : Sum  Inputs=+-+
  Transfer Fcn2 : TransferFcn  Numerator=[gnet]  Denominator=[1 gnet]
  Dobsv : Outport
  wires:
  Transfer Fcn2/1 -> Sum/2
  Sum8/1 -> Transfer Fcn2/1
  Derivative/1 -> Sum8/2, Gain/1
  Gain/1 -> Sum8/1, Sum/1
  Sum/1 -> Dobsv/1
  XRes/1 -> Derivative/1
  Acc./1 -> Sum8/3

== system BlockDiagram/CDOB/ND3/TimeDelayComp ==
  SysOut : Inport
  Dobsv : Inport  Port=2
  DelayCom : TransferFcn  Numerator=[a]  Denominator=[1 a 0]
  Sum8 : Sum  Inputs=|++
  FeedBack : Outport
  wires:
  DelayCom/1 -> Sum8/2
  SysOut/1 -> Sum8/1
  Sum8/1 -> FeedBack/1
  Dobsv/1 -> DelayCom/1

== system BlockDiagram/CDOB/ND4/CDOB1 ==
  XRes : Inport
  Acc. : Inport  Port=2
  Derivative : Derivative  CoefficientInTFapproximation=0
  Gain : Gain  Gain=gnet/a
  Sum : Sum  Inputs=-+|
  Sum8 : Sum  Inputs=+-+
  Transfer Fcn2 : TransferFcn  Numerator=[gnet]  Denominator=[1 gnet]
  Dobsv : Outport
  wires:
  Transfer Fcn2/1 -> Sum/2
  Sum8/1 -> Transfer Fcn2/1
  Derivative/1 -> Sum8/2, Gain/1
  Gain/1 -> Sum8/1, Sum/1
  Sum/1 -> Dobsv/1
  XRes/1 -> Derivative/1
  Acc./1 -> Sum8/3

== system BlockDiagram/CDOB/ND4/TimeDelayComp ==
  SysOut : Inport
  Dobsv : Inport  Port=2
  DelayCom : TransferFcn  Numerator=[a]  Denominator=[1 a 0]
  Sum8 : Sum  Inputs=|++
  FeedBack : Outport
  wires:
  DelayCom/1 -> Sum8/2
  SysOut/1 -> Sum8/1
  Sum8/1 -> FeedBack/1
  Dobsv/1 -> DelayCom/1

== system BlockDiagram/CDOB/ND5/CDOB1 ==
  XRes : Inport
  Acc. : Inport  Port=2
  Derivative : Derivative  CoefficientInTFapproximation=0
  Gain : Gain  Gain=gnet/a
  Sum : Sum  Inputs=-+|
  Sum8 : Sum  Inputs=+-+
  Transfer Fcn2 : TransferFcn  Numerator=[gnet]  Denominator=[1 gnet]
  Dobsv : Outport
  wires:
  Transfer Fcn2/1 -> Sum/2
  Sum8/1 -> Transfer Fcn2/1
  Gain/1 -> Sum8/1, Sum/1
  Sum/1 -> Dobsv/1
  XRes/1 -> Derivative/1
  Acc./1 -> Sum8/3
  Derivative/1 -> Gain/1, Sum8/2

== system BlockDiagram/CDOB/ND5/TimeDelayComp ==
  SysOut : Inport
  Dobsv : Inport  Port=2
  DelayCom : TransferFcn  Numerator=[a]  Denominator=[1 a 0]
  Sum8 : Sum  Inputs=|++
  FeedBack : Outport
  wires:
  DelayCom/1 -> Sum8/2
  SysOut/1 -> Sum8/1
  Sum8/1 -> FeedBack/1
  Dobsv/1 -> DelayCom/1
